simulink model "maglevAGH_LQI"  (R2020a)
settings: Solver=ode45  StartTime=0.0  StopTime=5  MaxStep=0.001  RelTol=1e-3  EnableMultiTasking=on
values from neighbouring files (symbols this model uses):
  g_E = 9.81    [identification_data.m]
  i_ep = sqrt(-2*m_b*g_E/L_d_ep)    [identification_data.m]
  K_lqi = lqr(Ai,Bi,Qi,Ri)    [identification_data.m]
  m_b = 58e-3    (= 0.058)    [identification_data.m]
  R_n = mean(R(1:end-1))    [identification_data.m]
  u_ep = R_n * i_ep    [identification_data.m]
  v_ep = 0    [identification_data.m]
  z_ep = 0.010    (= 0.01)    [identification_data.m]
undefined symbols (not defined in the file or in its folder): ind
settings Model: Creator=tutaj  LastModifiedBy=wkula
settings DataIOCC: LimitDataPoints=on  SaveFormat=Array  ReturnWorkspaceOutputs=off
settings OptimizationCC: LifeSpan=inf
settings DebuggingCC: UnderspecifiedInitializationDetection=Classic  MergeDetectMultiDrivingBlocksExec=none  SolverPrmCheckMsg=warning  StateNameClashWarn=warning  SFUnexpectedBacktrackingDiag=warning  SFNoUnconditionalDefaultTransitionDiag=warning  SFExecutionAtInitializationDiag=none  ArithmeticOperatorsInVariantConditions=warning
settings HardwareCC: ProdBitPerPointer=32  ProdBitPerSizeT=32  ProdBitPerPtrDiffT=32  ProdLargestAtomicFloat=None  ProdIntDivRoundTo=Undefined  ProdEndianess=Unspecified  ProdWordSize=32  ProdHWDeviceType=32-bit Generic
settings ModelReferenceCC: PropagateSignalLabelsOutOfModel=off
settings SFSimCC: SimUseLocalCustomCode=off  CustomCodeUndefinedFunction=UseInterfaceOnly
settings RTWCC: RTWUseLocalCustomCode=off
settings CodeAppCC: StateflowObjectComments=on
settings GRTTargetCC: TargetLangStandard=C89/C90 (ANSI)
settings ConfigComp: CovMetricSettings=dw  CovHtmlReporting=on  CovSaveCumulativeToWorkspaceVar=on  CovSaveSingleToWorkspaceVar=on  CovExternalEMLEnable=off

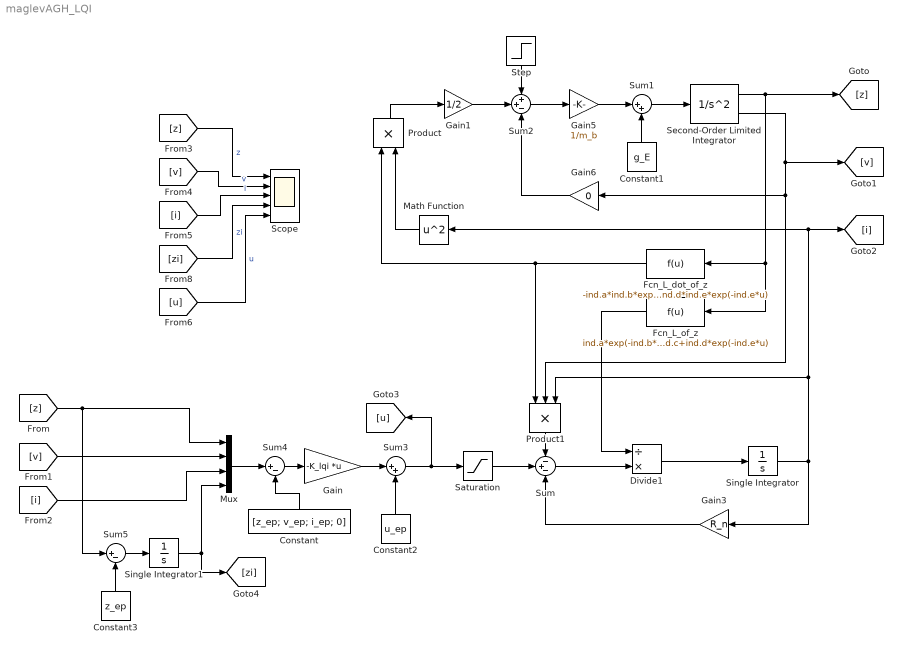
== system maglevAGH_LQI ==
  Constant : Constant  Value=[z_ep; v_ep; i_ep; 0]
  Constant1 : Constant  Value=g_E
  Constant2 : Constant  Value=u_ep
  Constant3 : Constant  Value=z_ep
  Divide1 : Product  Inputs=/*
  Fcn_L_dot_of_z : Fcn  Expr=-ind.a*ind.b*exp(-ind.b*u)-ind.d*ind.e*exp(-ind.e*u)
  Fcn_L_of_z : Fcn  Expr=ind.a*exp(-ind.b*u)+ind.c+ind.d*exp(-ind.e*u)
  Gain : Gain  Gain=-K_lqi  Multiplication=Matrix(K*u) (u vector)
  Gain1 : Gain  Gain=1/2
  Gain3 : Gain  Gain=R_n
  Gain5 : Gain  Gain=1/m_b
  Gain6 : Gain  Gain=0
  Math Function : Math  Operator=square  SignedPower=on  SaturateOnIntegerOverflow=on
  Mux : Mux
  Product : Product
  Product1 : Product  Inputs=3
  Saturation : Saturate  UpperLimit=12  LowerLimit=0
  Scope : Scope  NumInputPorts=5
  Second-Order Limited Integrator : SecondOrderIntegrator  ICX=z_ep - 0.0004  LimitX=on  UpperLimitX=0.2  LowerLimitX=0  ICDXDT=v_ep
  Single Integrator : Integrator  InitialCondition=i_ep
  Single Integrator1 : Integrator
  Step : Step  Time=2  After=0.02  SampleTime=0
  Sum : Sum  Inputs=-+-
  Sum1 : Sum  Inputs=|++
  Sum2 : Sum  Inputs=++-
  Sum3 : Sum  Inputs=|++
  Sum4 : Sum  Inputs=|+-
  Sum5 : Sum  Inputs=|+-
  wires:
  [z] -> Sum5/1, Mux/1
  [i] -> Mux/3
  Gain6/1 -> Sum2/3
  [z] -> Scope/1  "z"
  Gain/1 -> Sum3/1
  Constant3/1 -> Sum5/2
  [v] -> Scope/2  "v"
  Product1/1 -> Sum/1
  Single Integrator1/1 -> [zi], Mux/4
  Gain1/1 -> Sum2/2
  Gain5/1 -> Sum1/1
  Saturation/1 -> Sum/2
  [i] -> Scope/3  "i"
  [u] -> Scope/5  "u"
  [v] -> Mux/2
  Constant2/1 -> Sum3/2
  Constant/1 -> Sum4/2
  Mux/1 -> Sum4/1
  Sum2/1 -> Gain5/1
  Single Integrator/1 -> Gain3/1, [i], Math Function/1, Product1/3
  Constant1/1 -> Sum1/2
  Sum/1 -> Divide1/2
  Gain3/1 -> Sum/3
  Sum1/1 -> Second-Order Limited Integrator/1
  Second-Order Limited Integrator/1 -> [z], Fcn_L_of_z/1, Fcn_L_dot_of_z/1
  Second-Order Limited Integrator/2 -> [v], Product1/2, Gain6/1
  Math Function/1 -> Product/2
  Divide1/1 -> Single Integrator/1
  Step/1 -> Sum2/1
  [zi] -> Scope/4  "zi"
  Fcn_L_dot_of_z/1 -> Product/1, Product1/1
  Fcn_L_of_z/1 -> Divide1/1
  Sum5/1 -> Single Integrator1/1
  Product/1 -> Gain1/1
  Sum3/1 -> Saturation/1, [u]
  Sum4/1 -> Gain/1
